simulink model "flight_sim"  (R2017a)
settings: Solver=ode45  StartTime=0.0  StopTime=350  RelTol=1e-3
values from neighbouring files (symbols this model uses):
  g = 9.81    [parameters.m]
  gam_0 = pi/2    (= 1.57079632679)    [parameters.m]
  gam_in = 0.10    (= 0.1)    [parameters.m]
  h_0 = 0    [parameters.m]
  m_dot = 132    [parameters.m]
  m_zfw = m_pay + m_dry    (= 6360.7)    [parameters.m]
  R_E = 6371e3    (= 6371000)    [parameters.m]
  t_turn = 30.0    (= 30)    [parameters.m]
  v_0 = 0.01    [parameters.m]
  x_0 = 0    [parameters.m]
libraries: simulink x2, aerolibanim x1
settings Model: Creator=Nilay  LastModifiedBy=Nilay

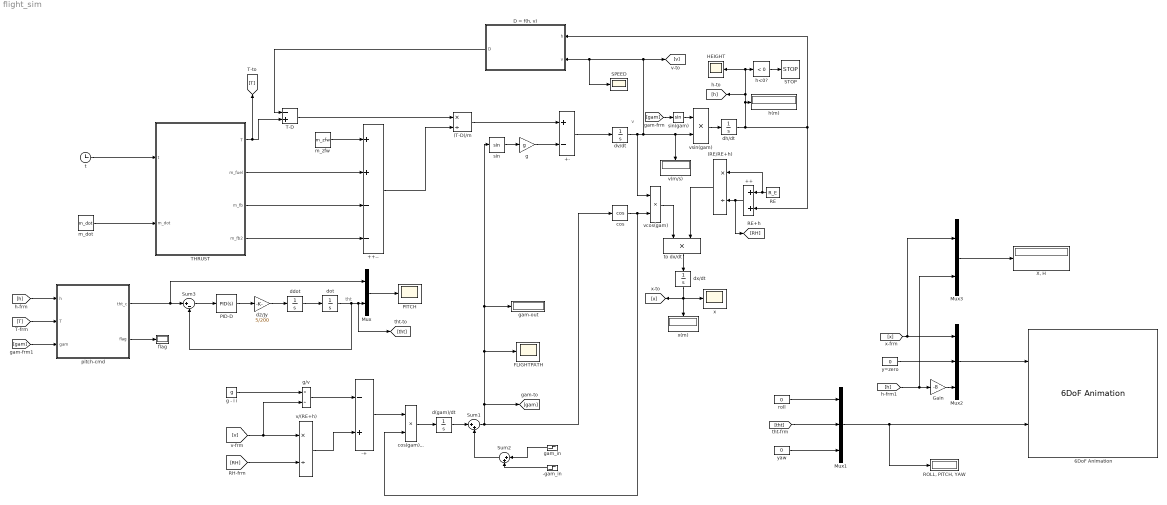
== system flight_sim ==
  note: tht
  note: v
  (RE/RE+h) : Product  Inputs=*/
  (T-D)/m : Product  Inputs=*/
  ++ : Sum
  ++-- : Sum  Inputs=++--
  +- : Sum  Inputs=+-
  -+ : Sum  Inputs=-+
  -gam_in : Step  Time=t_turn+1  Before=-gam_in  After=-gam_in  SampleTime=0
  6DoF Animation : aerolibanim/6DoF Animation  u1=[0 4000 -2000 2000 -5000 -3000]  u2=0.1  u3=1  u4=[4000 0 -5000]  u5=Fly alongside  u6=[0 2000 -2500]  u7=10  u8=on
      settings: SourceProductName=Aerospace Blockset
  "D = f(h, v)" : MATLAB Function  TreatAsAtomicUnit=on
  FLIGHTPATH : Scope
  Gain : Gain  Gain=-8
  HEIGHT : Scope
  Mux : Mux  Inputs=2
  Mux1 : Mux  Inputs=3
  Mux2 : Mux  Inputs=3
  Mux3 : Mux  Inputs=2
  PID-D : simulink/Continuous/PID Controller  Controller=PID  TimeDomain=Continuous-time  SampleTime=-1  IntegratorMethod=Forward Euler  FilterMethod=Forward Euler  Form=Parallel  UseFilter=on  ControllerParametersSource=internal  P=0  I=0  D=200/5  N=100  InitialConditionSource=internal  InitialConditionForIntegrator=0  InitialConditionForFilter=0  ExternalReset=none  LimitOutput=off  UpperSaturationLimit=inf  LowerSaturationLimit=-inf  LinearizeAsGain=on  AntiWindupMode=none  Kb=1  TrackingMode=off  Kt=1  PParamMin=[]  PParamMax=[]  IParamMin=[]  IParamMax=[]  DParamMin=[]  DParamMax=[]  NParamMin=[]  NParamMax=[]  KbParamMin=[]  KbParamMax=[]  KtParamMin=[]  KtParamMax=[]  POutMin=[]  POutMax=[]  IOutMin=[]  IOutMax=[]  DOutMin=[]  DOutMax=[]  NOutMin=[]  NOutMax=[]  KbOutMin=[]  KbOutMax=[]  KtOutMin=[]  KtOutMax=[]  IntegratorOutMin=[]  IntegratorOutMax=[]  FilterOutMin=[]  FilterOutMax=[]  SumOutMin=[]  SumOutMax=[]  SumI1OutMin=[]  SumI1OutMax=[]  SumI2OutMin=[]  SumI2OutMax=[]  SumI3OutMin=[]  SumI3OutMax=[]  SumDOutMin=[]  SumDOutMax=[]  SaturationOutMin=[]  SaturationOutMax=[]  IntegratorContinuousStateAttributes=''  IntegratorStateMustResolveToSignalObject=off  IntegratorRTWStateStorageClass=Auto  FilterContinuousStateAttributes=''  FilterStateMustResolveToSignalObject=off  FilterRTWStateStorageClass=Auto  DifferentiatorICPrevScaledInput=0  DifferentiatorOutMin=[]  DifferentiatorOutMax=[]  InitialConditionSetting=State (most efficient)
  PITCH : Scope
  RE : Constant  Value=R_E
  "ROLL, PITCH, YAW" : Display
  SPEED : Scope
  STOP : Stop
  Sum1 : Sum  Inputs=|++
  Sum2 : Sum  Inputs=|++
  Sum3 : Sum  Inputs=|+-
  T-D : Sum  Inputs=-+
  THRUST : MATLAB Function  TreatAsAtomicUnit=on
  "X, H" : Display
  cos : Trigonometry  Operator=cos
  cos(gam)... : Product
  d(gam)/dt : Integrator  InitialCondition=gam_0
  d2/Jy : Gain  Gain=5/200
  ddot : Integrator
  dh/dt : Integrator  InitialCondition=h_0
  dot : Integrator  InitialCondition=pi/2
  dv/dt : Integrator  InitialCondition=v_0
  dx/dt : Integrator  InitialCondition=x_0
  flag : Display
  g : Gain  Gain=g
  g - i i : Constant  Value=g
  g/v : Product  Inputs=*/
  gam-out : Display
  gam_in : Step  Time=t_turn  Before=gam_in  After=0  SampleTime=0
  h(m) : Display
  h<0? : simulink/Logic and Bit Operations/Compare To Zero  relop=<  OutDataTypeStr=boolean
  m_dot : Constant  Value=m_dot
  m_zfw : Constant  Value=m_zfw
  pitch-cmd : MATLAB Function  TreatAsAtomicUnit=on
  roll : Constant  Value=0
  sin : Trigonometry
  sin(gam) : Trigonometry
  t : Clock
  to dx/dt : Product
  v(m/s) : Display
  v/(RE+h) : Product  Inputs=*/
  vcos(gam) : Product
  vsin(gam) : Product
  x : Scope
  x(m) : Display
  y=zero : Constant  Value=0
  yaw : Constant  Value=0
  wires:
  t/1 -> THRUST/1(t)
  m_dot/1 -> THRUST/2(m_dot)
  THRUST/1(T) -> T-D/2, [T]
  m_zfw/1 -> ++--/1
  THRUST/3(m_fb) -> ++--/3
  THRUST/4(m_fb2) -> ++--/4
  THRUST/2(m_fuel) -> ++--/2
  T-D/1 -> (T-D)/m/1
  ++--/1 -> (T-D)/m/2
  (T-D)/m/1 -> +-/1
  g/1 -> +-/2
  sin/1 -> g/1
  +-/1 -> dv/dt/1
  dv/dt/1 -> vcos(gam)/1, v(m/s)/1, vsin(gam)/2, [v], SPEED/1, "D = f(h, v)"/2(v)
  vsin(gam)/1 -> dh/dt/1
  h<0?/1 -> STOP/1
  dh/dt/1 -> h<0?/1, HEIGHT/1, [h], h(m)/1, ++/2, "D = f(h, v)"/1(h)
  "D = f(h, v)"/1(D) -> T-D/1
  RE/1 -> (RE/RE+h)/1, ++/1
  ++/1 -> [RH], (RE/RE+h)/2
  (RE/RE+h)/1 -> to dx/dt/2
  to dx/dt/1 -> dx/dt/1
  dx/dt/1 -> [x], x(m)/1, x/1
  [v] -> g/v/2, v/(RE+h)/1
  [RH] -> v/(RE+h)/2
  g - i i/1 -> g/v/1
  g/v/1 -> -+/1
  v/(RE+h)/1 -> -+/2
  -+/1 -> cos(gam).../1
  cos(gam).../1 -> d(gam)/dt/1
  d(gam)/dt/1 -> Sum1/1
  Sum1/1 -> cos/1, FLIGHTPATH/1, gam-out/1, sin/1, [gam]
  cos/1 -> cos(gam).../2, vcos(gam)/2
  vcos(gam)/1 -> to dx/dt/1
  [gam] -> sin(gam)/1
  sin(gam)/1 -> vsin(gam)/1
  gam_in/1 -> Sum2/1
  -gam_in/1 -> Sum2/2
  Sum2/1 -> Sum1/2
  [h] -> pitch-cmd/1(h)
  [T] -> pitch-cmd/2(T)
  [gam] -> pitch-cmd/3(gam)
  pitch-cmd/2(flag) -> flag/1
  pitch-cmd/1(tht_c) -> Mux/1, Sum3/1
  Sum3/1 -> PID-D/1
  PID-D/1 -> d2/Jy/1
  d2/Jy/1 -> ddot/1
  ddot/1 -> dot/1
  dot/1 -> [tht], Mux/2, Sum3/2
  Mux/1 -> PITCH/1
  roll/1 -> Mux1/1
  [tht] -> Mux1/2
  yaw/1 -> Mux1/3
  Mux1/1 -> 6DoF Animation/2, "ROLL, PITCH, YAW"/1
  [x] -> Mux3/1, Mux2/1
  Mux2/1 -> 6DoF Animation/1
  y=zero/1 -> Mux2/2
  Gain/1 -> Mux2/3
  [h] -> Mux3/2, Gain/1
  Mux3/1 -> "X, H"/1

== matlab function flight_sim/pitch-cmd ==
  data: h input; tht_c output; T input; gam input; flag output
function [tht_c, flag] = fcn(h, T, gam)

persistent f

if isempty(f)
    f = 0;
end

if T<=0
    t_c = gam+pi;
    if t_c>pi
        t_c = pi;
    end
    f = 1;
elseif T<=0 && h <1000
    t_c = pi/2;
else
    t_c = gam;
end

flag = f;
tht_c = t_c;

== matlab function flight_sim/THRUST ==
  data: t input; T output; m_fuel output; m_fb output; m_fb2 output; m_dot input
function [T, m_fuel, m_fb, m_fb2] = fcn(t, m_dot)

persistent mfb
persistent mfb2

if isempty(mfb)
    mfb = 0;
end
if isempty(mfb2)
    mfb2 = 0;
end
mfuel = 21491.26;

if mfb <=0.65*mfuel
    THR = 346961.2;
    mfb = t*m_dot;
else
    THR = 0;
end

if (125<t) && (t<295)
    THR = -110000;
    mfb2 = (t-125)*(m_dot/3);
end

T = THR;
m_fb = mfb;
m_fb2 = mfb2;
m_fuel = mfuel;

== matlab function flight_sim/D = f(h, v) ==
  data: h input; D output; v input
function D = fcn(h, v)

CD = 0.075;
Di = 1.5;
A = pi*Di^2/4;

%density ISA model
if h <=11000
    T = 15.04 - 0.00649*h;
    p = 101.29*((T+273.1)/288.08)^5.258;
elseif (11000<h) &&(h<=25000)
    T = -56.46;
    p = 22.65*exp(1.73-0.000157*h);
else
    T = -131.21 + 0.00299*h;
    p = 2.488*((T+273.1)/216.6)^-11.388;
end

rho = p/(0.2869*(T+273.1));

%drag force D
Drag = 0.5*rho*v^2*A*CD;

D = Drag;
